simulink model "pde_sim"  (R2014a)
settings: Solver=ode45  StartTime=0.0  StopTime=3  RelTol=1e-3
values from neighbouring files (symbols this model uses):
  pde_sys = sys_class    [create_all_sys.m]
  sysr = ss(A_r,B_r,C_r,0)    [model_reduction.m]
undefined symbols (not defined in the file or in its folder): sysb, sysb_x0, syse, sysr_x0
settings Model: Creator=UX31  LastModifiedBy=UX31

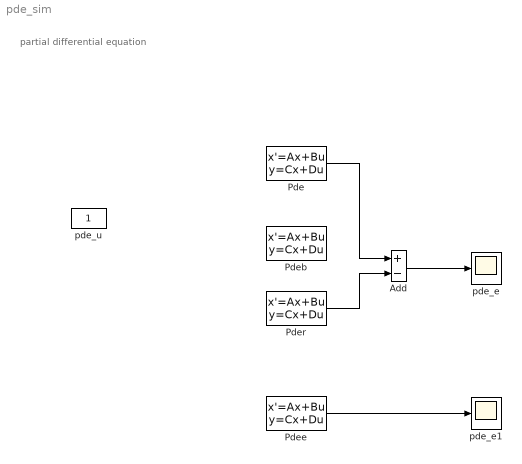
== system pde_sim ==
  note: partial differential equation
  Add : Sum  Inputs=+-
  Pde : StateSpace  A=pde_sys.sys.a  B=pde_sys.sys.b  C=pde_sys.sys.c  D=pde_sys.sys.d  X0=pde_sys.x0_lb
  Pdeb : StateSpace  A=sysb.sys.a  B=sysb.sys.b  C=sysb.sys.c  D=sysb.sys.d  X0=sysb_x0
  Pdee : StateSpace  A=syse.sys.a  B=syse.sys.b  C=syse.sys.c  D=syse.sys.d  X0=syse.x0_lb
  Pder : StateSpace  A=sysr.sys.a  B=sysr.sys.b  C=sysr.sys.c  D=sysr.sys.d  X0=sysr_x0
  pde_e : Scope
      settings: SaveName=ScopeData4
  pde_e1 : Scope
  pde_u : Constant
  wires:
  Add/1 -> pde_e/1
  Pdee/1 -> pde_e1/1
  Pder/1 -> Add/2
  Pde/1 -> Add/1
